simulink model "cx06_MA"  (Simulink 7.5)
settings: Solver=FixedStepDiscrete  StartTime=0.0  StopTime=10.0  RelTol=1e-3
undefined symbols (not defined in the file or in its folder): DiscIntNeverNeededParam, ECU555, int, motohawk_build_version, motohawk_trunc_name, motohawk_vardec_path
libraries: MotoHawk_lib x811, simulink x43, simulink_need_slupdate x1
(part 1 of 10)
settings Model: MotoHawkModelGUID=951679d1-661d-497d-a4-11-04-59-f9-a7-20  MotoHawkModelOpenTime=2017 12 11 19 53 57.471  MotoHawkBuildVersion=182  MotoHawkBuildStats=struct('TotalFLASH',{281968},'TotalEEPROM',{410},'TotalRAM',{20456},'AppFLASH',{75371},'AppEEPROM',{236},'AppRAM',{3912},'HeapRAM',{4096},'BuildSuccessCount',{137},'BuildErrorCount',{21},'OSRAM',{4768},'StackRAM',{7680},'FgndTimeStackSize',{3072},'FgndAngleStackSize',{0},'BgndStackSize',{2048},'IdleStackSize',{1024},'InterruptStackSize',{1536},'RTWBlockIOSize',{1884},'RTWDWorkSize',{428},'RTWPrevZCSize',{0},'VolatileSize',{468},'NonVolatileSize',{236},'ConstantSize',{1556},'NonVolatileFormatID',{54384})  MotoHawkModelSavedName=cx06_MA  MotoHawkModelElapsedTime=21020921.251  MotoHawkBuildGUID=fa4a9f3b-1218-4ceb-af-04-0c-06-13-21-16  MotoHawkBuildInfo=struct('model_name',{'cx06_MA'},'motohawk_version',{'2010a_sp1.49'},'motohawk_component_version',{'0.0.7'},'matlab_version',{'7.10.0'},'build_version',{'181'},'module_type',{'ECU555-80'},'layout_type',{'DEV'},'processor_family',{'PPC'},'processor_type',{'MPC555'},'toolchain_vendor',{'gcc-powerpc-eabi'},'toolchain_version',{'4.4.0'},'component',{0},'archive_file',{'PCM.a'},'enable_build',{1},'fptype',{0},'flash_size',{368640},'ee_size',{8192},'ram_size',{26624},'decram_size',{0},'module_memory_def',{'MPC555_ModMemoryDef_8KEE_Dev'},'eri_table0_rev',{9},'max_eri_table_size',{65535},'use_debug_vardecs',{1},'use_info_vardecs',{1},'fgnd_base_period_ms',{5},'bgnd_base_period_ms',{50},'root_build_dir',{'C:\Users\Owner\Documents\MATLAB\MoovadaCode2016\cx06_Updated_030317'},'build_dir',{'C:\Users\Owner\Documents\MATLAB\MoovadaCode2016\cx06_Updated_030317\cx06_MA_Build'},'dll_name',{'cx06_MA_181'},'srz_name',{'cx06_MA_181'},'fgnd_stack_size',{3072},'fgnd_angle_stack_size',{0},'bgnd_stack_size',{2048},'idle_stack_size',{1024},'irq_stack_size',{1536},'heap_size',{4096},'heap_margin',{409},'install_dll_dir',{'C:\ECUFiles\TDBDLL\'},'install_srz_dir',{'C:\ECUFiles\Programs\'},'app_int_stack_size',{1024},'shutdown_stack_size',{1024},'mingw_dir',{'C:\PROGRA~2\Woodward\DEVELO~1\TOOLCH~1\GCC\win32-pe\4_4_0\'},'motohawk_dir',{'C:\PROGRA~2\Woodward\MCS\MotoHawk\2010A_~1.49'},'toolchain_dir',{'C:\Program Files (x86)\Woodward\DevelopmentTools\Toolchains\GCC\powerpc-eabi\4_4_0\'},'matlab_root',{'C:\Program Files (x86)\MATLAB\R2010a'},'model_guid',{'951679d1-661d-497d-a4-11-04-59-f9-a7-20'},'build_guid',{'fa4a9f3b-1218-4ceb-af-04-0c-06-13-21-16'},'token_guid',{'no token'})  Creator=LanD  LastModifiedBy=Owner
settings OptimizationCC: InlineParams=on  InitFltsAndDblsToZero=on  OptimizeModelRefInitCode=on  LifeSpan=1
settings DebuggingCC: SolverPrmCheckMsg=none  InheritedTsInSrcMsg=none  TasksWithSamePriorityMsg=none  StrictBusMsg=Warning
settings HardwareCC: ProdEndianess=BigEndian  ProdHWDeviceType=Specified
settings RTWCC: SystemTargetFile=motohawk_ert_rtw.tlc  TLCOptions="-aCustomNonFinites=\"motohawk_genrtnonfinite.tlc\""  MakeCommand=motohawk_make_rtw  TemplateMakefile=motohawk_ert_rtw.tmf  Description=MotoHawk(tm) Rapid Prototyping  ProcessScript=motohawk_ert_rtw_make_rtw_hook
settings CodeAppCC: IgnoreCustomStorageClasses=off  MaxIdLength=100  CustomSymbolStrField=$H$N$M
settings STFCustomTargetCC: ModelReferenceCompliant=off  CombineOutputUpdateFcns=on  ERTCustomFileBanners=on  SupportContinuousTime=off  SupportNonInlinedSFcns=off  SystemTargetFile=motohawk_ert_rtw.tlc
settings ERTTargetCC: MultiwordLength=2048  ModelReferenceCompliant=off  ParMdlRefBuildCompliant=off  CompOptLevelCompliant=off  ERTFirstTimeCompliant=off  ModelStepFunctionPrototypeControlCompliant=off  CPPClassGenCompliant=off  ERTCustomFileTemplate=example_file_process.tlc  ConvertIfToSwitch=off

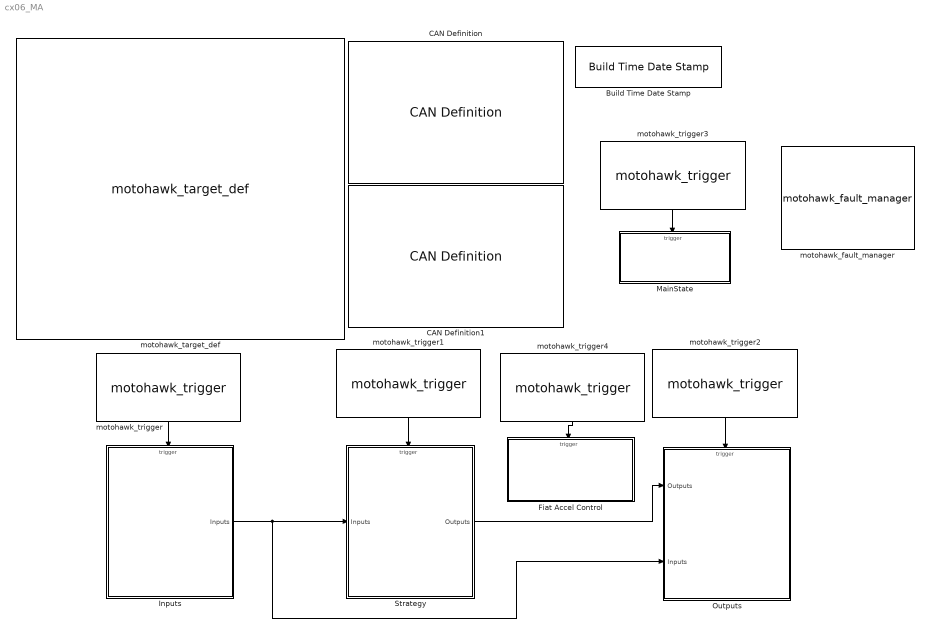
== system cx06_MA ==
  Build Time Date Stamp : MotoHawk_lib/Extra Development Blocks/Build Time Date Stamp  SystemSampleTime=-1
  CAN Definition : MotoHawk_lib/CAN Blocks/CAN Definition  Priority=-100  nam=['CAN_' num2str(1)]  text_resource=CAN1  code_resource=NONE  val_resource=-1  target=ECU555-80  bus=-2  btime=500 kbaud  pre=1  prop=0  pseg1=0  pseg2=0  resyn=0  tx_queue_size=16  rx_queue_size=16  use_protocol=on  city_id=hex2dec('B')  access_level=4  mototune_group='System | System Config | Communication Config'
  CAN Definition1 : MotoHawk_lib/CAN Blocks/CAN Definition  Priority=-100  nam=['CAN_' num2str(2)]  text_resource=CAN2  code_resource=NONE  val_resource=-1  target=ECU555-80  bus=-2  btime=500 kbaud  pre=1  prop=0  pseg1=0  pseg2=0  resyn=0  tx_queue_size=16  rx_queue_size=16  use_protocol=off  city_id=hex2dec('B')  access_level=4  mototune_group='System | System Config | Communication Config'
  Fiat Accel Control : Subsystem  TreatAsAtomicUnit=on
  Inputs : Subsystem  TreatAsAtomicUnit=on
  MainState : Subsystem  AncestorBlock=MotoHawk_lib/Extra Development Blocks/Main Power Relay/Background
      settings: RTWSystemCode=Function  RTWFcnNameOpts=Use subsystem name  RTWFileNameOpts=Use function name
  Outputs : Subsystem  TreatAsAtomicUnit=on
      settings: RTWSystemCode=Function  RTWFcnNameOpts=Use subsystem name  RTWFileNameOpts=Use function name
  Strategy : Subsystem  TreatAsAtomicUnit=on
      settings: RTWSystemCode=Function  RTWFcnNameOpts=Use subsystem name  RTWFileNameOpts=Use function name
  motohawk_fault_manager : MotoHawk_lib/Fault Management Blocks/motohawk_fault_manager  storage=FLASH  read_level=1  write_level=1  clear_level=1  xytype=uint8  mototune_group='Faults'
  motohawk_target_def : MotoHawk_lib/motohawk_target_def  Priority=-65535  target=ECU555-80  layout=DEV  fptype=single (32 bits)  fgnd_stack_size=3*1024  fgnd_angle_stack_size=0  bgnd_stack_size=2*1024  idle_stack_size=1024  irq_stack_size=1536  app_int_stack_size=1024  shutdown_stack_size=1024  heap_size=4*1024  show_margins=off  fgnd_stack_margin=(3*1024) * 0.1  fgnd_angle_stack_margin=0  bgnd_stack_margin=(2*1024) * 0.1  idle_stack_margin=(1024) * 0.1  irq_stack_margin=(1536) * 0.1  app_int_stack_margin=(1024) * 0.1  shutdown_stack_margin=(1024) * 0.1  heap_margin=(4*1024) * 0.1  comp_name=bdroot  comp_img='KVASER_CAN_USB.jpg'  comp_security=No Encryption  comp_build_pass='mhbuild'  comp_sim_pass='mhsim'  comp_multi=off  show_filenames=off  dll_name=motohawk_trunc_name(bdroot, ['_' motohawk_build_version], 13)  srz_name=motohawk_trunc_name(bdroot, ['_' motohawk_build_version], 50)  build_dir=''  comp_dir='.'
  motohawk_trigger : MotoHawk_lib/Trigger Blocks/motohawk_trigger  Tag=Trigger  trigger=FGND_RTI_PERIODIC  function_name=Trigger_FGND_RTI_PERIODIC_6445p0006  priority_order=0  inherited=off  run_disabled=off  override_app_monitor=off  target=ECU555_80
  motohawk_trigger1 : MotoHawk_lib/Trigger Blocks/motohawk_trigger  Tag=Trigger  trigger=FGND_RTI_PERIODIC  function_name=Trigger_FGND_RTI_PERIODIC_6445p0005  priority_order=0  inherited=off  run_disabled=off  override_app_monitor=off  target=ECU555_80
  motohawk_trigger2 : MotoHawk_lib/Trigger Blocks/motohawk_trigger  Tag=Trigger  trigger=FGND_RTI_PERIODIC  function_name=Trigger_FGND_RTI_PERIODIC_6445p0004  priority_order=0  inherited=off  run_disabled=off  override_app_monitor=off  target=ECU555_80
  motohawk_trigger3 : MotoHawk_lib/Trigger Blocks/motohawk_trigger  Tag=Trigger  Priority=255  trigger=BGND_BASE_PERIODIC  function_name=Trigger_BGND_BASE_PERIODIC_6445p0002  priority_order=255  inherited=on  run_disabled=on  override_app_monitor=off  target=ECU555_80
  motohawk_trigger4 : MotoHawk_lib/Trigger Blocks/motohawk_trigger  Tag=Trigger  trigger=FGND_RTI_PERIODIC  function_name=Trigger_FGND_RTI_PERIODIC_6445p0001  priority_order=0  inherited=off  run_disabled=off  override_app_monitor=off  target=ECU555_80
  wires:
  motohawk_trigger/1 -> Inputs/Trigger
  motohawk_trigger1/1 -> Strategy/Trigger
  motohawk_trigger2/1 -> Outputs/Trigger
  Inputs/1(Inputs) -> Strategy/1(Inputs), Outputs/2(Inputs)
  Strategy/1(Outputs) -> Outputs/1(Outputs)
  motohawk_trigger3/1 -> MainState/Trigger
  motohawk_trigger4/1 -> Fiat Accel Control/Trigger

== system cx06_MA/Fiat Accel Control ==
  function : TriggerPort  TriggerType=function-call
  Data Type Conversion{,1..3} (4 alike) : DataTypeConversion  OutDataType=sfix(16)  OutScaling=2^0
  Discrete-Time Integrator : DiscreteIntegrator  SampleTime=-1  OutDataType=sfix(16)  OutScaling=2^0  LimitOutput=on  UpperSaturationLimit=1  LowerSaturationLimit=0  ICPrevOutput=DiscIntNeverNeededParam  ICPrevScaledInput=DiscIntNeverNeededParam
  Discrete-Time Integrator1 : DiscreteIntegrator  SampleTime=-1  OutDataType=sfix(16)  OutScaling=2^0  LimitOutput=on  UpperSaturationLimit=1  LowerSaturationLimit=0  ICPrevOutput=DiscIntNeverNeededParam  ICPrevScaledInput=DiscIntNeverNeededParam
  Gain : Gain  Gain=5/1023  ParameterDataType=sfix(16)  ParameterScaling=2^0  OutDataType=sfix(16)  OutScaling=2^0
  Gain1 : Gain  Gain=5/1023  ParameterDataType=sfix(16)  ParameterScaling=2^0  OutDataType=sfix(16)  OutScaling=2^0
  Gain2 : Gain  Gain=4096/5  ParameterDataType=sfix(16)  ParameterScaling=2^0  OutDataType=int(16)  OutScaling=2^0  RndMeth=Nearest
  Gain3 : Gain  Gain=4096/5  ParameterDataType=sfix(16)  ParameterScaling=2^0  OutDataType=int(16)  OutScaling=2^0  RndMeth=Nearest
  Product{,1..3} (4 alike) : Product  OutDataType=sfix(16)  OutScaling=2^0  RndMeth=Zero
  Saturation : Saturate  UpperLimit=5  LowerLimit=0
  Saturation1 : Saturate  UpperLimit=5  LowerLimit=0
  Sum : Sum  Inputs=|+-  OutDataType=sfix(16)  OutScaling=2^0
  Sum1 : Sum  Inputs=|+-  OutDataType=sfix(16)  OutScaling=2^0
  Sum2 : Sum  OutDataType=sfix(16)  OutScaling=2^0
  Sum3 : Sum  OutDataType=sfix(16)  OutScaling=2^0
  motohawk_ain : MotoHawk_lib/Analog I//O Blocks/motohawk_ain  res_name=[]  text_resource=AN11M  code_resource=NONE  val_resource=-1  target=ECU555-80  resource_enum_str=(None)=-1,ECUP=53,DRVP=54,XDRP=55,AN1M=56,AN2M=57,AN3M=58,AN4M=59,AN5M=60,AN6M=61,AN7M=62,AN8M=63,AN9M=64,AN10M=65,AN11M=66,AN12M=67,AN13M=68,AN14M=69,AN15M=70,AN16M=71,AN17M=72,AN18M=73,AN19M=74,O2A=90,O2B=91,XDRP_B=92  altref=5V Reference  typ=uint16  num_adc_bits=10  use_stat=off  use_vardec=off  nam='AIN'  read_level=1  write_level=1  group='System | I/O Pins | Inputs Config'
  motohawk_ain1 : MotoHawk_lib/Analog I//O Blocks/motohawk_ain  res_name=[]  text_resource=AN10M  code_resource=NONE  val_resource=-1  target=ECU555-80  resource_enum_str=(None)=-1,ECUP=53,DRVP=54,XDRP=55,AN1M=56,AN2M=57,AN3M=58,AN4M=59,AN5M=60,AN6M=61,AN7M=62,AN8M=63,AN9M=64,AN10M=65,AN11M=66,AN12M=67,AN13M=68,AN14M=69,AN15M=70,AN16M=71,AN17M=72,AN18M=73,AN19M=74,O2A=90,O2B=91,XDRP_B=92  altref=5V Reference  typ=uint16  num_adc_bits=10  use_stat=off  use_vardec=off  nam='AIN'  read_level=1  write_level=1  group='System | I/O Pins | Inputs Config'
  motohawk_calibration1 : MotoHawk_lib/Calibration & Probing Blocks/motohawk_calibration  nam='volt_out_1'  val=0  storage=Calibration  show_more=on  name_source=Use Parameter  data_type=double  read_level=1  write_level=1  ovr_cals=on  view_as=Number  enum_struct={'Disabled', 'Enabled'}  vector_style=Wide Row  use_help_units=off  help=''  units=''  use_header_enum=off  row_header_enum={}  col_header_enum={}  use_min_max=on  min_val=0  max_val=5  use_precision=off  precision=''  gain=1  offset=0  exp=1  use_mototune_group=off  mototune_group=motohawk_vardec_path(gcb)
  motohawk_calibration2 : MotoHawk_lib/Calibration & Probing Blocks/motohawk_calibration  nam='volt_out_2'  val=0  storage=Calibration  show_more=on  name_source=Use Parameter  data_type=Inherit from 'Default Value'  read_level=1  write_level=1  ovr_cals=on  view_as=Number  enum_struct={'Disabled', 'Enabled'}  vector_style=Wide Row  use_help_units=off  help=''  units=''  use_header_enum=off  row_header_enum={}  col_header_enum={}  use_min_max=on  min_val=0  max_val=5  use_precision=off  precision=''  gain=1  offset=0  exp=1  use_mototune_group=off  mototune_group=motohawk_vardec_path(gcb)
  motohawk_calibration3 : MotoHawk_lib/Calibration & Probing Blocks/motohawk_calibration  nam='Kp'  val=0  storage=Calibration  show_more=on  name_source=Use Parameter  data_type=double  read_level=1  write_level=1  ovr_cals=on  view_as=Number  enum_struct={'Disabled', 'Enabled'}  vector_style=Wide Row  use_help_units=off  help=''  units=''  use_header_enum=off  row_header_enum={}  col_header_enum={}  use_min_max=on  min_val=0  max_val=5  use_precision=off  precision=''  gain=1  offset=0  exp=1  use_mototune_group=off  mototune_group=motohawk_vardec_path(gcb)
  motohawk_calibration4 : MotoHawk_lib/Calibration & Probing Blocks/motohawk_calibration  nam='Ki'  val=0  storage=Calibration  show_more=on  name_source=Use Parameter  data_type=double  read_level=1  write_level=1  ovr_cals=on  view_as=Number  enum_struct={'Disabled', 'Enabled'}  vector_style=Wide Row  use_help_units=off  help=''  units=''  use_header_enum=off  row_header_enum={}  col_header_enum={}  use_min_max=on  min_val=0  max_val=5  use_precision=off  precision=''  gain=1  offset=0  exp=1  use_mototune_group=off  mototune_group=motohawk_vardec_path(gcb)
  motohawk_calibration5 : MotoHawk_lib/Calibration & Probing Blocks/motohawk_calibration  nam='PWM_Freq'  val=150000  storage=Calibration  show_more=on  name_source=Use Parameter  data_type=Inherit from 'Default Value'  read_level=1  write_level=1  ovr_cals=on  view_as=Number  enum_struct={'Disabled', 'Enabled'}  vector_style=Wide Row  use_help_units=off  help=''  units=''  use_header_enum=off  row_header_enum={}  col_header_enum={}  use_min_max=on  min_val=200  max_val=200000  use_precision=off  precision=''  gain=1  offset=0  exp=1  use_mototune_group=off  mototune_group=motohawk_vardec_path(gcb)
  motohawk_override_abs : MotoHawk_lib/Calibration & Probing Blocks/motohawk_override_abs  SystemSampleTime=-1  parent_name='duty_override'  parent_val=0  show_more=off  name_source=Use Parameter  parent_read_level=1  parent_override_level=1  view_as=Number  enum_struct={'Disabled', 'Enabled'}  use_help_units=off  parent_help=''  parent_units=''  use_min_max=off  parent_min=-inf  parent_max=inf  use_precision=off  parent_precision=''  parent_gain=1  parent_offset=0  parent_exp=1  use_mototune_group=off  parent_group=motohawk_vardec_path(gcb)
  motohawk_probe1 : MotoHawk_lib/Calibration & Probing Blocks/motohawk_probe  nam='effect'  show_more=on  name_source=Use Parameter  read_level=1  view_as=Number  enum_struct={'Disabled', 'Enabled'}  vector_style=Wide Row  use_help_units=off  help=''  units=''  use_header_enum=off  row_header_enum={}  col_header_enum={}  use_precision=on  precision='3.3'  gain=1  offset=0  exp=1  use_mototune_group=off  mototune_group=motohawk_vardec_path(gcb)
  motohawk_probe2 : MotoHawk_lib/Calibration & Probing Blocks/motohawk_probe  nam='error'  show_more=on  name_source=Use Parameter  read_level=1  view_as=Number  enum_struct={'Disabled', 'Enabled'}  vector_style=Wide Row  use_help_units=off  help=''  units=''  use_header_enum=off  row_header_enum={}  col_header_enum={}  use_precision=on  precision='3.3'  gain=1  offset=0  exp=1  use_mototune_group=off  mototune_group=motohawk_vardec_path(gcb)
  motohawk_probe3 : MotoHawk_lib/Calibration & Probing Blocks/motohawk_probe  nam='duty'  show_more=on  name_source=Use Parameter  read_level=1  view_as=Number  enum_struct={'Disabled', 'Enabled'}  vector_style=Wide Row  use_help_units=off  help=''  units=''  use_header_enum=off  row_header_enum={}  col_header_enum={}  use_precision=on  precision='3.3'  gain=1  offset=0  exp=1  use_mototune_group=off  mototune_group=motohawk_vardec_path(gcb)
  motohawk_probe4 : MotoHawk_lib/Calibration & Probing Blocks/motohawk_probe  nam='ain'  show_more=on  name_source=Use Parameter  read_level=1  view_as=Number  enum_struct={'Disabled', 'Enabled'}  vector_style=Wide Row  use_help_units=off  help=''  units=''  use_header_enum=off  row_header_enum={}  col_header_enum={}  use_precision=on  precision='3.3'  gain=1  offset=0  exp=1  use_mototune_group=off  mototune_group=motohawk_vardec_path(gcb)
  motohawk_probe5 : MotoHawk_lib/Calibration & Probing Blocks/motohawk_probe  nam='Ipart'  show_more=on  name_source=Use Parameter  read_level=1  view_as=Number  enum_struct={'Disabled', 'Enabled'}  vector_style=Wide Row  use_help_units=off  help=''  units=''  use_header_enum=off  row_header_enum={}  col_header_enum={}  use_precision=on  precision='3.3'  gain=1  offset=0  exp=1  use_mototune_group=off  mototune_group=motohawk_vardec_path(gcb)
  motohawk_probe6 : MotoHawk_lib/Calibration & Probing Blocks/motohawk_probe  nam='Ppart'  show_more=on  name_source=Use Parameter  read_level=1  view_as=Number  enum_struct={'Disabled', 'Enabled'}  vector_style=Wide Row  use_help_units=off  help=''  units=''  use_header_enum=off  row_header_enum={}  col_header_enum={}  use_precision=on  precision='3.3'  gain=1  offset=0  exp=1  use_mototune_group=off  mototune_group=motohawk_vardec_path(gcb)
  motohawk_pwm : MotoHawk_lib/Analog I//O Blocks/motohawk_pwm  res_name=[]  text_resource=FINJ5  code_resource=NONE  val_resource=-1  target=ECU555-80  resource_enum_str=(None)=-1,FUELP=0,ETC=1,HSOL1=2,HSOL2=3,HSOL3=4,HSOL4=5,START=6,OILP=11,FINJ1=12,FINJ2=13,FINJ3=14,FINJ4=15,FINJ5=16,FINJ6=17,AINJ1=18,AINJ2=19,AINJ3=20,AINJ4=21,AINJ5=22,AINJ6=23,TACH=24,EST 1=36,EST 2=37,EST 3=38,EST 4=39,EST 5=40,EST 6=41,EST 7=42,EST 8=43  freq_mode=-1  min_freq=2  use_max_freq=off  max_freq=42949672.96  use_enable=off  use_brake=off  output_current=off  output_fault_status=off  use_child=off  use_vardec=off  nam='PWM'  read_level=1  write_level=1  group='System | I/O Pins | Outputs Config'
  motohawk_pwm1 : MotoHawk_lib/Analog I//O Blocks/motohawk_pwm  res_name=[]  text_resource=AINJ5  code_resource=NONE  val_resource=-1  target=ECU555-80  resource_enum_str=(None)=-1,FUELP=0,ETC=1,HSOL1=2,HSOL2=3,HSOL3=4,HSOL4=5,START=6,OILP=11,FINJ1=12,FINJ2=13,FINJ3=14,FINJ4=15,FINJ5=16,FINJ6=17,AINJ1=18,AINJ2=19,AINJ3=20,AINJ4=21,AINJ5=22,AINJ6=23,TACH=24,EST 1=36,EST 2=37,EST 3=38,EST 4=39,EST 5=40,EST 6=41,EST 7=42,EST 8=43  freq_mode=-1  min_freq=2  use_max_freq=off  max_freq=42949672.96  use_enable=off  use_brake=off  output_current=off  output_fault_status=off  use_child=off  use_vardec=off  nam='PWM'  read_level=1  write_level=1  group='System | I/O Pins | Outputs Config'
  wires:
  motohawk_calibration2/1 -> Sum1/1
  motohawk_ain/1 -> Gain1/1
  motohawk_calibration1/1 -> Sum/1
  motohawk_ain1/1 -> Gain/1, motohawk_probe4/1
  Sum1/1 -> Discrete-Time Integrator1/1, Product3/2
  motohawk_calibration3/1 -> Product1/2, Product3/1
  Sum/1 -> Discrete-Time Integrator/1, Product1/1, motohawk_probe2/1
  Discrete-Time Integrator/1 -> Product/1, motohawk_probe5/1
  motohawk_calibration4/1 -> Product/2, Product2/1
  Discrete-Time Integrator1/1 -> Product2/2
  Product/1 -> Sum3/1
  Product1/1 -> Sum3/2, motohawk_probe6/1
  Product2/1 -> Sum2/1
  Product3/1 -> Sum2/2
  motohawk_calibration5/1 -> Data Type Conversion2/1, Data Type Conversion3/1
  Sum2/1 -> Saturation1/1
  Sum3/1 -> Saturation/1, motohawk_probe1/1
  Gain/1 -> Sum/2
  Gain1/1 -> Sum1/2
  Saturation/1 -> Gain2/1
  Gain2/1 -> Data Type Conversion/1
  Gain3/1 -> Data Type Conversion1/1
  Saturation1/1 -> Gain3/1
  Data Type Conversion1/1 -> motohawk_pwm1/1
  Data Type Conversion/1 -> motohawk_override_abs/1
  Data Type Conversion2/1 -> motohawk_pwm1/2
  Data Type Conversion3/1 -> motohawk_pwm/2
  motohawk_override_abs/1 -> motohawk_pwm/1, motohawk_probe3/1

== system cx06_MA/Inputs ==
  note: GMLAN
  function : TriggerPort  TriggerType=function-call
  Analog Inputs : Subsystem
  Bus Creator : BusCreator  Inputs=7
  Drive-by-Wire CAN Input : Subsystem
  Fiat CAN Input : Subsystem
  GMLAN Inputs : Subsystem
  IPT CAN Input : Subsystem
  JCI CAN Input : Subsystem
  Urea Inputs : Subsystem
  Inputs : Outport  OutDataType=sfix(16)  OutScaling=2^0
  wires:
  IPT CAN Input/1(IPT) -> Bus Creator/1  "IPT"
  JCI CAN Input/1(JCI) -> Bus Creator/2  "JCI"
  Fiat CAN Input/1(FIAT) -> Bus Creator/3  "Fiat"
  GMLAN Inputs/1(GMLAN) -> Bus Creator/5
  Analog Inputs/1(Analog) -> Bus Creator/6  "Analog"
  Urea Inputs/1(Urea) -> Bus Creator/7  "Urea"
  Drive-by-Wire CAN Input/1(AO) -> Bus Creator/4  "AO"
  Bus Creator/1 -> Inputs/1

== system cx06_MA/MainState ==
  note: MainState
      | 0 - PowerUp
      | 1 - Run
      | 2 - Estop
      | 3 - PowerDown
      | 4 - Shutdown
  note: Control Main Power Relay
  f : TriggerPort  TriggerType=function-call  ZeroCross=off
  Call Startup Event : Subsystem
  Chart : Stateflow chart  TreatAsAtomicUnit=on
  Constant : Constant  OutDataTypeMode=uint8  OutDataType=sfix(16)  OutScaling=2^0  OutDataTypeStr=uint8
  Constant1 : Constant  Value=100  OutDataTypeMode=uint16  OutDataType=sfix(16)  OutScaling=2^0  OutDataTypeStr=uint16
  Display Variable Event Function-Call : MotoHawk_lib/Extra Development Blocks/Display Variable Event Function-Call  SystemSampleTime=-1  nam='RestoreNVFactoryDefaults'  level=1  enum_str={'Run', 'Restore To Defaults'}  help_str='Restores NonVolatile Memory to Factory Defaults'  group='System | NonVolatile Storage'
  Display Variable Event Function-Call1 : MotoHawk_lib/Extra Development Blocks/Display Variable Event Function-Call  SystemSampleTime=-1  nam='StoreNV'  level=1  enum_str={'Run', 'Store To EEPROM'}  help_str='Stores RAM-Shadowed memory to serial EEPROM'  group='System | NonVolatile Storage'
  Gain : Gain  Gain=12.21/2.21*5/1023  ParameterDataType=sfix(16)  ParameterScaling=2^0  OutDataTypeMode=Specify via dialog  OutDataType=float('single')  OutDataTypeStr=float('single')
  Logical Operator : Logic  Operator=XOR  AllPortsSameDT=off  OutDataTypeMode=boolean  OutDataTypeStr=boolean
  Logical Operator3 : Logic  Operator=OR  OutDataTypeMode=boolean  OutDataTypeStr=boolean
  Post Shutdown two ticks before MPRD off : Subsystem
  Relational Operator : RelationalOperator  LogicOutDataTypeMode=boolean  OutDataTypeStr=boolean  ZeroCross=off  InputSameDT=on
  Save NV Vars one tick before MPRD off : Subsystem
  Shutdown power on ECU565-128 : Subsystem
  Terminator : Terminator
  Unit Delay1 : UnitDelay  SampleTime=-1
  Unit Delay2 : UnitDelay  SampleTime=-1
  motohawk_ain1 : MotoHawk_lib/Analog I//O Blocks/motohawk_ain  res_name=[]  text_resource=DRVP  code_resource=RES_ECUP  val_resource=-1  target=ECU555-80  resource_enum_str=(None)=-1,ECUP=53,DRVP=54,XDRP=55,AN1M=56,AN2M=57,AN3M=58,AN4M=59,AN5M=60,AN6M=61,AN7M=62,AN8M=63,AN9M=64,AN10M=65,AN11M=66,AN12M=67,AN13M=68,AN14M=69,AN15M=70,AN16M=71,AN17M=72,AN18M=73,AN19M=74,O2A=90,O2B=91,XDRP_B=92  altref=5V Reference  typ=uint16  num_adc_bits=10  use_stat=on  use_vardec=off  nam='AIN'  read_level=1  write_level=1  group='System | I/O Pins | Inputs Config'
  motohawk_ain5 : MotoHawk_lib/Analog I//O Blocks/motohawk_ain  res_name=[]  text_resource=ECUP  code_resource=RES_ECUP  val_resource=-1  target=ECU555-80  resource_enum_str=(None)=-1,ECUP=53,DRVP=54,XDRP=55,AN1M=56,AN2M=57,AN3M=58,AN4M=59,AN5M=60,AN6M=61,AN7M=62,AN8M=63,AN9M=64,AN10M=65,AN11M=66,AN12M=67,AN13M=68,AN14M=69,AN15M=70,AN16M=71,AN17M=72,AN18M=73,AN19M=74,O2A=90,O2B=91,XDRP_B=92  altref=5V Reference  typ=uint16  num_adc_bits=10  use_stat=on  use_vardec=off  nam='AIN'  read_level=1  write_level=1  group='System | I/O Pins | Inputs Config'
  motohawk_calibration : MotoHawk_lib/Calibration & Probing Blocks/motohawk_calibration  nam='ESTOP_Invert'  val=1  storage=Calibration  show_more=on  name_source=Use Parameter  data_type=uint8  read_level=1  write_level=1  ovr_cals=on  view_as=Enumeration  enum_struct={'False', 'True'}  vector_style=Wide Row  use_help_units=off  help=''  units=''  use_header_enum=off  row_header_enum={}  col_header_enum={}  use_min_max=off  min_val=-inf  max_val=inf  use_precision=off  precision=''  gain=1  offset=0  exp=1  use_mototune_group=off  mototune_group=motohawk_vardec_path(gcb)
  motohawk_data_def : MotoHawk_lib/Data Storage Blocks/motohawk_data_def  nam='mainState'  container_nam=''  data=0  typ=uint8  struct_nam='MyStruct'  storage=Volatile  outputRef=off  use_vardec=on  window=Display  read_level=1  write_level=1  ovr_cals=on  view_as=Enumeration  enum_struct={'PowerUp', 'Run', 'EStop', 'PowerDown', 'Shutdown'}  vector_style=Wide Row  use_help_units=on  help=''  units=''  use_header_enum=off  row_header_enum=''  col_header_enum=''  use_min_max=off  min_val=-inf  max_val=inf  use_precision=off  precision=''  gain=1  offset=0  exp=1  use_mototune_group=off  mototune_group=motohawk_vardec_path(gcb)  eval_name=mainState  data_stores=motohawk_sfun_data_def_data_stores  struct_instances=motohawk_sfun_data_def_struct_instances  vardecs=motohawk_sfun_data_def_vardecs
  motohawk_data_write : MotoHawk_lib/Data Storage Blocks/motohawk_data_write  source=Lookup By Name  structure=Scalar  operation=Write scalar into location by index  sz_vec=-1  sz_row=3  sz_col=2  typ=uint8  nam='mainState'  checkNull=on  write_read_only=off  struct_inst_name='Struct1'  struct_name='MyStruct'
  motohawk_din : MotoHawk_lib/Digital I//O Blocks/motohawk_din  resource_name='ESTOP'  text_resource=ESTOP  code_resource=RES_AN1M  val_resource=-1  target=ECU555-80  resource_enum_str=(None)=-1,AN1M=56,AN2M=57,AN3M=58,AN4M=59,AN5M=60,AN6M=61,AN7M=62,AN8M=63,AN9M=64,AN10M=65,AN11M=66,AN12M=67,AN13M=68,AN14M=69,AN15M=70,AN16M=71,AN17M=72,AN18M=73,AN19M=74,O2A=90,O2B=91,DG1M=93,DG2M=94,DG4M=96,ESTOP=97  pullup=Weak  use_stat=off  use_vardec=on  nam='ESTOP'  read_level=1  write_level=1  group='I/O Pins | Inputs Config'
  motohawk_dout : MotoHawk_lib/Digital I//O Blocks/motohawk_dout  text_resource=MPRD  code_resource=NONE  val_resource=-1  target=ECU555-80  resource_enum_str=(None)=-1,FUELP=0,HSOL1=2,HSOL2=3,HSOL3=4,HSOL4=5,START=6,OILP=11,FINJ1=12,FINJ2=13,FINJ3=14,FINJ4=15,FINJ5=16,FINJ6=17,AINJ1=18,AINJ2=19,AINJ3=20,AINJ4=21,AINJ5=22,AINJ6=23,TACH=24,EST 1=36,EST 2=37,EST 3=38,EST 4=39,EST 5=40,EST 6=41,EST 7=42,EST 8=43,MPRD=52  use_diag=off  use_vardec=off  nam='DOUT'  read_level=1  write_level=1  group='System | I/O Pins | Outputs Config'
  motohawk_override_abs : MotoHawk_lib/Calibration & Probing Blocks/motohawk_override_abs  SystemSampleTime=-1  parent_name='MPRD'  parent_val=0  show_more=on  name_source=Use Parameter  parent_read_level=1  parent_override_level=1  view_as=Enumeration  enum_struct={'Off', 'On'}  use_help_units=off  parent_help='Directly Override Main Power Relay'  parent_units='boolean'  use_min_max=on  parent_min=0  parent_max=1  use_precision=off  parent_precision=''  parent_gain=1  parent_offset=0  parent_exp=1  use_mototune_group=on  parent_group=motohawk_vardec_path(gcb)
  motohawk_probe : MotoHawk_lib/Calibration & Probing Blocks/motohawk_probe  nam='EStop_Cal'  show_more=off  name_source=Use Parameter  read_level=1  view_as=Number  enum_struct={'Disabled', 'Enabled'}  vector_style=Wide Row  use_help_units=off  help=''  units=''  use_header_enum=off  row_header_enum={}  col_header_enum={}  use_precision=off  precision=''  gain=1  offset=0  exp=1  use_mototune_group=off  mototune_group=motohawk_vardec_path(gcb)
  motohawk_probe1 : MotoHawk_lib/Calibration & Probing Blocks/motohawk_probe  nam='In_EStop'  show_more=on  name_source=Use Parameter  read_level=1  view_as=Number  enum_struct={'Disabled', 'Enabled'}  vector_style=Wide Row  use_help_units=off  help=''  units=''  use_header_enum=off  row_header_enum={}  col_header_enum={}  use_precision=off  precision=''  gain=1  offset=0  exp=1  use_mototune_group=on  mototune_group='Debug | Inputs'
  motohawk_probe2 : MotoHawk_lib/Calibration & Probing Blocks/motohawk_probe  nam='ECUP_Raw'  show_more=on  name_source=Use Parameter  read_level=1  view_as=Number  enum_struct={'Disabled', 'Enabled'}  vector_style=Wide Row  use_help_units=off  help=''  units=''  use_header_enum=off  row_header_enum={}  col_header_enum={}  use_precision=on  precision=''  gain=1  offset=0  exp=1  use_mototune_group=off  mototune_group=motohawk_vardec_path(gcb)
  motohawk_probe3 : MotoHawk_lib/Calibration & Probing Blocks/motohawk_probe  nam='In_ECUP'  show_more=on  name_source=Use Parameter  read_level=1  view_as=Number  enum_struct={'Disabled', 'Enabled'}  vector_style=Wide Row  use_help_units=off  help=''  units=''  use_header_enum=off  row_header_enum={}  col_header_enum={}  use_precision=off  precision=''  gain=1  offset=0  exp=1  use_mototune_group=on  mototune_group='Debug | Inputs'
  motohawk_probe4 : MotoHawk_lib/Calibration & Probing Blocks/motohawk_probe  nam='DRVP_Raw'  show_more=on  name_source=Use Parameter  read_level=1  view_as=Number  enum_struct={'Disabled', 'Enabled'}  vector_style=Wide Row  use_help_units=off  help=''  units=''  use_header_enum=off  row_header_enum={}  col_header_enum={}  use_precision=on  precision=''  gain=1  offset=0  exp=1  use_mototune_group=off  mototune_group=motohawk_vardec_path(gcb)
  motohawk_probe5 : MotoHawk_lib/Calibration & Probing Blocks/motohawk_probe  nam='DRVP_Cal'  show_more=on  name_source=Use Parameter  read_level=1  view_as=Number  enum_struct={'Disabled', 'Enabled'}  vector_style=Wide Row  use_help_units=off  help=''  units=''  use_header_enum=off  row_header_enum={}  col_header_enum={}  use_precision=on  precision='2.1'  gain=1  offset=0  exp=1  use_mototune_group=off  mototune_group=motohawk_vardec_path(gcb)
  motohawk_restore_nvmem : MotoHawk_lib/Data Storage Blocks/motohawk_restore_nvmem  SystemSampleTime=-1
  motohawk_store_nvmem : MotoHawk_lib/Data Storage Blocks/motohawk_store_nvmem  SystemSampleTime=-1
  wires:
  Logical Operator3/1 -> motohawk_override_abs/1
  Display Variable Event Function-Call1/1 -> motohawk_store_nvmem/Trigger
  Display Variable Event Function-Call/1 -> motohawk_restore_nvmem/Trigger
  Unit Delay2/1 -> Logical Operator3/2
  Unit Delay1/1 -> Unit Delay2/1, Shutdown power on ECU565-128/Trigger
  Constant1/1 -> Relational Operator/2
  motohawk_ain5/1 -> Relational Operator/1, motohawk_probe2/1
  motohawk_override_abs/1 -> motohawk_dout/1
  Chart/2(MPRD) -> Logical Operator3/1
  Chart/3(Shutdown) -> Unit Delay1/1, Save NV Vars one tick before MPRD off/Trigger
  Relational Operator/1 -> Chart/2(Ecup)
  Constant/1 -> Chart/3(PowerDown_Cmplt)
  Chart/1(MS_State) -> motohawk_data_write/1
  Chart/4(PowerUp) -> Call Startup Event/Trigger
  Chart/5(PowerDown) -> Post Shutdown two ticks before MPRD off/Trigger
  motohawk_ain5/2 -> motohawk_probe3/1
  motohawk_calibration/1 -> Logical Operator/1
  motohawk_din/1 -> Logical Operator/2
  Logical Operator/1 -> motohawk_probe/1, Chart/1(EStop), motohawk_probe1/1
  motohawk_ain1/1 -> motohawk_probe4/1, Gain/1
  Gain/1 -> motohawk_probe5/1
  motohawk_ain1/2 -> Terminator/1

== system cx06_MA/Outputs ==
  Outputs : Inport  OutDataType=sfix(16)  OutScaling=2^0
  Inputs : Inport  Port=2  OutDataType=sfix(16)  OutScaling=2^0
  function : TriggerPort  TriggerType=function-call
  ARDAQ Outputs : Subsystem
  Analog Outputs : Subsystem
  Debug Outputs : Subsystem
  Drive-by-Wire CAN Output : Subsystem
  Fiat CAN Output : Subsystem
  GMLAN Outputs : Subsystem
  IPT CAN Output : Subsystem
  JCI CAN Output : Subsystem
  wires:
  Outputs/1 -> IPT CAN Output/1(Outputs), Drive-by-Wire CAN Output/1(Outputs), GMLAN Outputs/1(Outputs), Analog Outputs/1(Outputs), Debug Outputs/1(Outputs)
  Inputs/1 -> IPT CAN Output/2(Inputs), GMLAN Outputs/2(Inputs), Analog Outputs/2(Inputs), Debug Outputs/2(In1), ARDAQ Outputs/1(In1), Fiat CAN Output/1(Inputs)

== system cx06_MA/Strategy ==
  Inputs : Inport  OutDataType=sfix(16)  OutScaling=2^0
  function : TriggerPort  TriggerType=function-call
  A/C Control Code : Subsystem
  Bus Creator : BusCreator
  Fiat/GMLAN Control Code : Subsystem
  Hybrid Control Code : Subsystem
  Unit Delay : UnitDelay  SampleTime=-1
  Urea Control Code : Subsystem
  Outputs : Outport  OutDataType=sfix(16)  OutScaling=2^0
  wires:
  Inputs/1 -> Urea Control Code/1(In1), Fiat/GMLAN Control Code/1(In1), A/C Control Code/1(In1), Hybrid Control Code/1(Inputs)
  Hybrid Control Code/1(Outputs) -> Bus Creator/2  "Hybrid"
  Urea Control Code/1(Out) -> Bus Creator/3  "Urea"
  Fiat/GMLAN Control Code/1(Out1) -> Bus Creator/4  "Fiat/GMLAN"
  Bus Creator/1 -> Outputs/1
  Hybrid Control Code/2(Warn_Eng_Kill) -> Unit Delay/1
  Unit Delay/1 -> Urea Control Code/2(Warn_Eng_Kill)
  A/C Control Code/1(Out1) -> Bus Creator/1  "AC"

== system cx06_MA/Inputs/Analog Inputs ==
  AC_Pres : Subsystem
  Bus Creator : BusCreator  Inputs=6
  Cruise Buttons : Subsystem
  Driver Inputs : Subsystem
  Fuel Level : Subsystem
  MAF : Subsystem
  Trans Inputs : Subsystem
  Analog : Outport  OutDataType=sfix(16)  OutScaling=2^0
  wires:
  Driver Inputs/1(Driver) -> Bus Creator/2  "Driver"
  Trans Inputs/1(Trans) -> Bus Creator/3  "Trans"
  Bus Creator/1 -> Analog/1
  Cruise Buttons/1(Cruise_Button) -> Bus Creator/1  "cruiseBut"
  Fuel Level/1(Fuel_Level) -> Bus Creator/4  "Fuel_Level"
  AC_Pres/1(AC_Pres) -> Bus Creator/5  "AC_Pres"
  MAF/1(MAF) -> Bus Creator/6  "MAF"

== system cx06_MA/Inputs/Drive-by-Wire CAN Input ==
  Bus Creator : BusCreator  Inputs=2
  Compare To Constant1 : simulink/Logic and Bit Operations/Compare To Constant  SystemSampleTime=-1  relop=>  const=30  LogicOutDataTypeMode=boolean  ZeroCross=off
  Compare To Constant2 : simulink/Logic and Bit Operations/Compare To Constant  SystemSampleTime=-1  relop=>  const=30  LogicOutDataTypeMode=boolean  ZeroCross=off
  Read CAN Message : MotoHawk_lib/CAN Blocks/Read CAN Message  nam=['CAN_' num2str(1)]  bus=-2  msg=CANRx_AO_369  queue=1  slot=''  valid=off  stale=on  labelwires=on
  Read CAN Message1 : MotoHawk_lib/CAN Blocks/Read CAN Message  nam=['CAN_' num2str(1)]  bus=-2  msg=CANRx_AO_370  queue=1  slot=''  valid=off  stale=on  labelwires=on
  motohawk_fault_def1 : MotoHawk_lib/Fault Management Blocks/motohawk_fault_def  nam='CAN2AO370'  mode=Enabled - Persistent  id=[]  x=10  y=11  input_suspected=on  indeterminate=off  increment_xy=on  downsample_count=1  ovr_cals=on  ovr_actions=on  show_actions=on  action1_name='inhibitDiesel'  action1_cond=Active  action2_name=''  action2_cond=(None)  action3_name=''  action3_cond=(None)  action4_name=''  action4_cond=(None)
  motohawk_fault_def2 : MotoHawk_lib/Fault Management Blocks/motohawk_fault_def  nam='CAN2AO369'  mode=Enabled - Persistent  id=[]  x=10  y=11  input_suspected=on  indeterminate=off  increment_xy=on  downsample_count=1  ovr_cals=on  ovr_actions=on  show_actions=on  action1_name='inhibitDiesel'  action1_cond=Active  action2_name=''  action2_cond=(None)  action3_name=''  action3_cond=(None)  action4_name=''  action4_cond=(None)
  motohawk_probe{,1..3} (4 alike) : MotoHawk_lib/Calibration & Probing Blocks/motohawk_probe  nam='Probe'  show_more=on  name_source=Use Input Wire Name  read_level=1  view_as=Number  enum_struct={'Disabled', 'Enabled'}  vector_style=Wide Row  use_help_units=off  help=''  units=''  use_header_enum=off  row_header_enum={}  col_header_enum={}  use_precision=off  precision=''  gain=1  offset=0  exp=1  use_mototune_group=off  mototune_group=motohawk_vardec_path(gcb)
  AO : Outport  OutDataType=sfix(16)  OutScaling=2^0
  wires:
  Bus Creator/1 -> AO/1
  Compare To Constant2/1 -> motohawk_fault_def2/1  "AgeCount"
  Read CAN Message/1 -> Compare To Constant2/1  "AgeCount"
  Read CAN Message/2 -> motohawk_probe/1  "CAN_EWARN1"
  Read CAN Message/3 -> motohawk_probe1/1, Bus Creator/1  "Output1_V"
  Compare To Constant1/1 -> motohawk_fault_def1/1  "AgeCount"
  Read CAN Message1/1 -> Compare To Constant1/1  "AgeCount"
  Read CAN Message1/2 -> motohawk_probe2/1  "CAN_EWARN2"
  Read CAN Message1/3 -> motohawk_probe3/1, Bus Creator/2  "Output2_V"
